simulink model "sim_track6"  (Simulink 5.0)
settings: Solver=ode45  StartTime=0.0  StopTime=Tmax  RelTol=1e-6
undefined symbols (not defined in the file or in its folder): dF, dFo, dG, dK, dQ, dQu, dR, nF, nFo, nG, nK, nQ, nQu, nR, T, tauF, tauG, tauQ, tauQu, tauR
settings Model: LastModifiedBy=Administrator  BlockReductionOpt=off  BooleanDataType=off  RTWOptions="-aEnforceIntegerDowncast=1 -aFoldNonRolledExpr=1 -aInlineInvariantSignals=1 -aInlineParameters=0 -aLocalBlockOutputs=1 -aRollThreshold=5 -aGenerateReport=0 -aGenCodeOnly=0 -aRTWVerbose=1 -aIncludeHyperlinkInReport=0 -aLaunchReport=0 -aForceParamTrailComments=0 -aGenerateComments=1 -aIgnoreCustomStorageClasses=1 -aIncHierarchyInIds=0 -aMaxRTWIdLen=31 -aShowEliminatedStatements=0 -aPrefixModelToSubsysFcnNames=1 -aIncDataTypeInIds=0 -aInsertBlockDesc=0 -aSimulinkBlockComments=1 -aInlinedPrmAccess=\"Literals\"  -aSuppressErrorStatus=0 -aModelReferenceCompliant=1 -aSupportNonInlinedSFcns=1 -aSupportContinuousTime=1 -aSupportComplex=1 -aSupportNonFinite=1 -aSupportAbsoluteTime=1 -aTargetPreCompLibLocation=\"\" -aTargetLibSuffix=\"\" -aTargetFcnLib=\"ansi_tfl_tmw.mat\" -aMultiInstanceERTCode=0 -aLogVarNameModifier=\"rt_\" -aIsPILTarget=0 -aCombineOutputUpdateFcns=0 -aGenerateASAP2=0 -aGenerateSampleERTMain=0 -aGenerateFullHeader=1 -aUtilityFuncGeneration=\"Auto\" -aIncludeFileDelimiter=\"Auto\" -aIncludeMdlTerminateFcn=1 -aPurelyIntegerCode=0 -aERTCustomFileBanners=0 -aRTWCAPIStates=0 -aRTWCAPIParams=0 -aRTWCAPISignals=0 -aMatFileLogging=1 -aGenFloatMathFcnCalls=\"ANSI_C\" -aExtModeMexFile=\"ext_comm\" -aExtModeTransport=0 -aExtModeStaticAllocSize=1000000 -aExtModeTesting=0 -aExtModeStaticAlloc=0 -aExtMode=0  -aInitFltsAndDblsToZero=1 -aInitFltsAndDblsToZero=1"

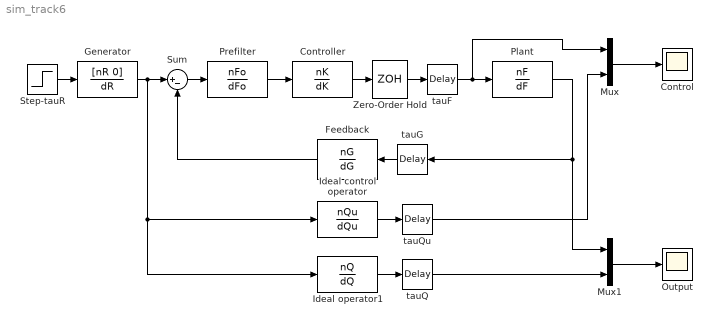
== system sim_track6 ==
  Control : Scope
      settings: TimeRange=10  YMin=0  YMax=2.1  SaveName=u  DataFormat=Array
  Controller : DiscreteTransferFcn  Numerator=nK  Denominator=dK  SampleTime=T
  Feedback : TransferFcn  Orientation=left  Numerator=nG  Denominator=dG
  Generator : TransferFcn  Numerator=[nR 0]  Denominator=dR
  Ideal control operator : TransferFcn  Numerator=nQu  Denominator=dQu
  Ideal operator1 : TransferFcn  Numerator=nQ  Denominator=dQ
  Mux : Mux  Inputs=2
  Mux1 : Mux  Inputs=2
  Output : Scope
      settings: TimeRange=50  YMin=0  YMax=14  SaveName=y  DataFormat=Array
  Plant : TransferFcn  Numerator=nF  Denominator=dF
  Prefilter : TransferFcn  Numerator=nFo  Denominator=dFo
  Step-tauR : Step  Time=tauR
  Sum : Sum  Inputs=|+-  SaturateOnIntegerOverflow=on  InputSameDT=on
  Zero-Order Hold : ZeroOrderHold  SampleTime=T
  tauF : TransportDelay  DelayTime=tauF  BufferSize=10240
  tauG : TransportDelay  Orientation=left  DelayTime=tauG  BufferSize=10240
  tauQ : TransportDelay  DelayTime=tauQ  BufferSize=10240
  tauQu : TransportDelay  DelayTime=tauQu  BufferSize=10240
  wires:
  Plant/1 -> Mux1/1, tauG/1
  Step-tauR/1 -> Generator/1
  Mux/1 -> Control/1
  Mux1/1 -> Output/1
  Ideal control operator/1 -> tauQu/1
  tauQu/1 -> Mux/2
  Ideal operator1/1 -> tauQ/1
  tauQ/1 -> Mux1/2
  Prefilter/1 -> Controller/1
  Controller/1 -> Zero-Order Hold/1
  Zero-Order Hold/1 -> tauF/1
  tauF/1 -> Mux/1, Plant/1
  Sum/1 -> Prefilter/1
  tauG/1 -> Feedback/1
  Feedback/1 -> Sum/2
  Generator/1 -> Sum/1, Ideal operator1/1, Ideal control operator/1
